simulink model "real_vedio"  (R2021b)
settings: Solver=FixedStepDiscrete  StartTime=0.0  StopTime=100  RelTol=1e-3
PreLoadFcn:
  | n=8; %Number of quantization bits
undefined symbols (not defined in the file): gray, IsPositionTracked, IsSkeletonTracked, JointDepthIndices, JointImageIndices, JointTrackingState, JointWorldCoordinates, none, PositionDepthIndices, PositionImageIndices, PositionWorldCoordinates, Rec, SDTV, SegmentationData, SkeletonTrackingID, videoinput
libraries: commdigbbndpm3 x6, commutil2 x6, dspsigattribs x6, commchan3 x3, visionconversions x2, imaqlib x1
settings Model: Creator=magarini  LastModifiedBy=mluser
settings SolverCC: AlgebraicLoopSolver=TrustRegion
settings DataIOCC: LimitDataPoints=on  SaveFormat=Array  SignalLoggingSaveFormat=ModelDataLogs  ReturnWorkspaceOutputs=off
settings OptimizationCC: BlockReduction=off  ConditionallyExecuteInputs=off  DefaultParameterBehavior=Inlined  ExpressionDepthLimit=2147483647  LifeSpan=inf
settings DebuggingCC: AlgebraicLoopMsg=error  UnderspecifiedInitializationDetection=Classic  MergeDetectMultiDrivingBlocksExec=none  SolverPrmCheckMsg=warning  MultiTaskCondExecSysMsg=warning  MultiTaskRateTransMsg=warning  SingleTaskRateTransMsg=warning  FcnCallInpInsideContextMsg=warning  StateNameClashWarn=warning  SFUnexpectedBacktrackingDiag=warning  SFNoUnconditionalDefaultTransitionDiag=warning  SFExecutionAtInitializationDiag=none  SFMachineParentedDataDiag=warning  ArithmeticOperatorsInVariantConditions=warning
settings HardwareCC: ProdBitPerPointer=32  ProdBitPerSizeT=32  ProdBitPerPtrDiffT=32  ProdLargestAtomicFloat=None  ProdIntDivRoundTo=Undefined  ProdEndianess=Unspecified  ProdWordSize=32  ProdHWDeviceType=ASIC/FPGA->ASIC/FPGA  ProdEqTarget=off
settings ModelReferenceCC: PropagateSignalLabelsOutOfModel=off
settings SFSimCC: SimUseLocalCustomCode=off  SimParseCustomCode=off  CustomCodeUndefinedFunction=UseInterfaceOnly
settings RTWCC: RTWUseLocalCustomCode=off
settings CodeAppCC: StateflowObjectComments=on
settings GRTTargetCC: TargetLangStandard=C89/C90 (ANSI)  CombineOutputUpdateFcns=off  GRTInterface=on
settings ConfigComp: CovMetricSettings=dw  CovSaveCumulativeToWorkspaceVar=on  CovSaveSingleToWorkspaceVar=on  CovExternalEMLEnable=off  CovSFcnEnable=off

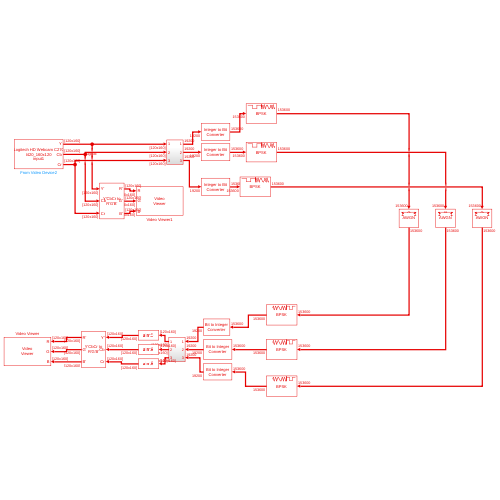
[thumbnail: Simulink's stored preview of the top-level diagram]
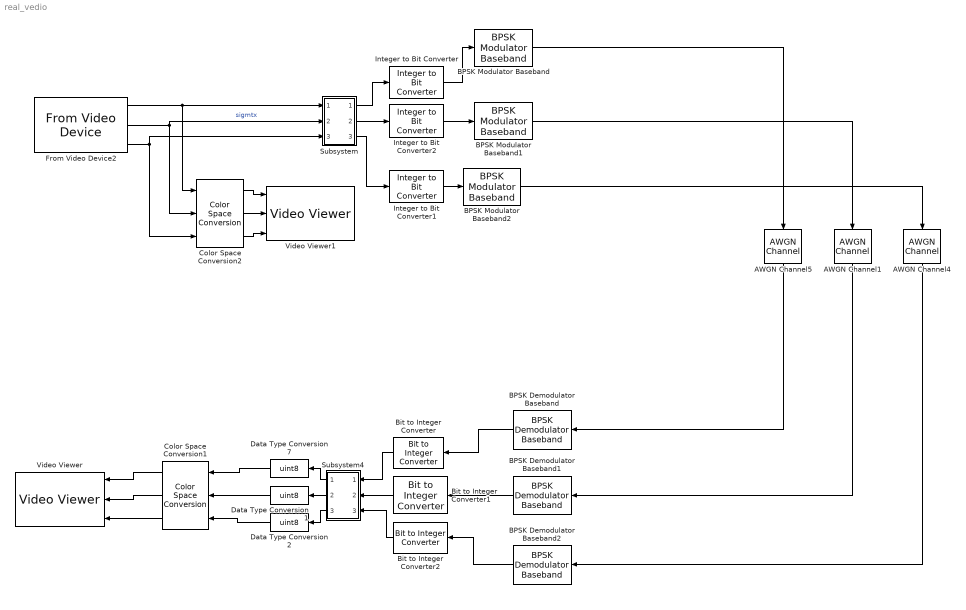
== system real_vedio ==
  AWGN Channel1 : commchan3/AWGN Channel  InputProcessing=Columns as channels (frame based)  seed=67  noiseMode="Signal to noise ratio  (Eb/No)"  EbNodB=10  EsNodB=10  SNRdB=10  bitsPerSym=1  Ps=1  Tsym=1  variance=1
  AWGN Channel4 : commchan3/AWGN Channel  InputProcessing=Columns as channels (frame based)  seed=67  noiseMode="Signal to noise ratio  (Eb/No)"  EbNodB=10  EsNodB=10  SNRdB=10  bitsPerSym=1  Ps=1  Tsym=1  variance=1
  AWGN Channel5 : commchan3/AWGN Channel  InputProcessing=Columns as channels (frame based)  seed=67  noiseMode="Signal to noise ratio  (Eb/No)"  EbNodB=10  EsNodB=10  SNRdB=10  bitsPerSym=1  Ps=1  Tsym=1  variance=1
  BPSK Demodulator Baseband : commdigbbndpm3/BPSK Demodulator Baseband  DecType=Hard decision  VarSource=Dialog  Variance=1  Ph=0  outDtype=Inherit via internal rule  derotateFactorWordLen=16  derotateFactorDataTypeStr=Inherit: Same word length as input  derotateFactorLastDataTypeStr=Inherit: Same word length as input
  BPSK Demodulator Baseband1 : commdigbbndpm3/BPSK Demodulator Baseband  DecType=Hard decision  VarSource=Dialog  Variance=1  Ph=0  outDtype=Inherit via internal rule  derotateFactorWordLen=16  derotateFactorDataTypeStr=Inherit: Same word length as input  derotateFactorLastDataTypeStr=Inherit: Same word length as input
  BPSK Demodulator Baseband2 : commdigbbndpm3/BPSK Demodulator Baseband  DecType=Hard decision  VarSource=Dialog  Variance=1  Ph=0  outDtype=Inherit via internal rule  derotateFactorWordLen=16  derotateFactorDataTypeStr=Inherit: Same word length as input  derotateFactorLastDataTypeStr=Inherit: Same word length as input
  BPSK Modulator Baseband : commdigbbndpm3/BPSK Modulator Baseband  Ph=0  outDtype=double  outWordLen=16  outUDDataType=sfix(16)  outFracLenMode=Best precision  outFracLen=15  outDataTypeStr=double  outLastDataTypeStr=double
  BPSK Modulator Baseband1 : commdigbbndpm3/BPSK Modulator Baseband  Ph=0  outDtype=double  outWordLen=16  outUDDataType=sfix(16)  outFracLenMode=Best precision  outFracLen=15  outDataTypeStr=double  outLastDataTypeStr=double
  BPSK Modulator Baseband2 : commdigbbndpm3/BPSK Modulator Baseband  Ph=0  outDtype=double  outWordLen=16  outUDDataType=sfix(16)  outFracLenMode=Best precision  outFracLen=15  outDataTypeStr=double  outLastDataTypeStr=double
  Bit to Integer Converter : commutil2/Bit to Integer Converter  nbits=8  bitOrder=MSB first  signedOutputValues=Unsigned  outDtype=Inherit via internal rule  outDtypeSigned=Inherit via internal rule
  Bit to Integer Converter1 : commutil2/Bit to Integer Converter  nbits=8  bitOrder=MSB first  signedOutputValues=Unsigned  outDtype=Inherit via internal rule  outDtypeSigned=Inherit via internal rule
  Bit to Integer Converter2 : commutil2/Bit to Integer Converter  nbits=8  bitOrder=MSB first  signedOutputValues=Unsigned  outDtype=Inherit via internal rule  outDtypeSigned=Inherit via internal rule
  Color Space Conversion1 : visionconversions/Color Space  Conversion  conversion=Obsolete  conversionActive=Y'CbCr to R'G'B'  wp_str=D65  rec=Rec. 601 (SDTV)  sys=1125/60/2:1  imagePorts=Separate color signals
  Color Space Conversion2 : visionconversions/Color Space  Conversion  conversion=Obsolete  conversionActive=Y'CbCr to R'G'B'  wp_str=D65  rec=Rec. 601 (SDTV)  sys=1125/60/2:1  imagePorts=Separate color signals
  Data Type Conversion1 : DataTypeConversion  OutDataTypeStr=uint8
  Data Type Conversion2 : DataTypeConversion  OutDataTypeStr=uint8
  Data Type Conversion7 : DataTypeConversion  OutDataTypeStr=uint8
  From Video Device2 : imaqlib/From Video Device  DeviceMenu=INPUTDEVS  Device=winvideo 1 (Logitech HD Webcam C270)  ObjConstructor=videoinput('winvideo', 1)  VideoFormatMenu=INPUTFORMATS  VideoFormat=I420_160x120  VideoSource=input1  ROIPosition=[0 0 120 160]  EnableHWTrigger=off  TriggerConfiguration=none/none  SampleTime=1/25  OutputPortsMode=Separate color signals  DataType=uint8  CanDoHWTrigger=no  ReturnedColorSpace=YCbCr  BlockHandle=5600.0004  ROIWidth=160  ROIHeight=120  ROIColumn=0  ROIRow=0  EngXMLPath=/MATLAB/toolbox/imaq/imaq/private  DevXMLPath=C:\MATLAB\SupportPackages\R2015a\osgenericvideointerface\toolbox\imaq\supportpackages\genericvideo\adaptor\win64  EngLibPath=/MATLAB/toolbox/imaq/imaqblks/imaqmex/glnxa64  ColorSpace=YCbCr  BayerSensorAlignment=grbg  AllMetadata=IsPositionTracked;IsSkeletonTracked;JointDepthIndices;JointImageIndices;JointTrackingState;JointWorldCoordinates;PositionDepthIndices;PositionImageIndices;PositionWorldCoordinates;SegmentationData;SkeletonTrackingID  ImaqMode=off
  Integer to Bit Converter : commutil2/Integer to Bit Converter  nbits=8  signedInputValues=Unsigned  bitOrder=MSB first  outDtype=Inherit via internal rule
  Integer to Bit Converter1 : commutil2/Integer to Bit Converter  nbits=8  signedInputValues=Unsigned  bitOrder=MSB first  outDtype=Inherit via internal rule
  Integer to Bit Converter2 : commutil2/Integer to Bit Converter  nbits=8  signedInputValues=Unsigned  bitOrder=MSB first  outDtype=Inherit via internal rule
  Subsystem : Subsystem
  Subsystem4 : Subsystem
  Video Viewer : VideoViewer  imagePorts=separate color signals  colormapValue=gray(256)  FigPos=[502 1000 410 300]
  Video Viewer1 : VideoViewer  imagePorts=separate color signals  colormapValue=gray(256)  FigPos=[65 1007 410 300]
  wires:
  Color Space Conversion1/1 -> Video Viewer/1
  Color Space Conversion1/2 -> Video Viewer/2
  Color Space Conversion1/3 -> Video Viewer/3
  Color Space Conversion2/1 -> Video Viewer1/1
  Color Space Conversion2/2 -> Video Viewer1/2
  Color Space Conversion2/3 -> Video Viewer1/3
  From Video Device2/2 -> Subsystem/2(In2), Color Space Conversion2/2  "sigmtx"
  From Video Device2/3 -> Subsystem/3(In3), Color Space Conversion2/3
  Subsystem/1(Out1) -> Integer to Bit Converter/1
  Subsystem/2(Out2) -> Integer to Bit Converter2/1
  Subsystem/3(Out3) -> Integer to Bit Converter1/1
  From Video Device2/1 -> Subsystem/1(In1), Color Space Conversion2/1
  Subsystem4/1(Out1) -> Data Type Conversion7/1
  Subsystem4/2(Out2) -> Data Type Conversion1/1
  Subsystem4/3(Out3) -> Data Type Conversion2/1
  BPSK Demodulator Baseband/1 -> Bit to Integer Converter/1
  BPSK Demodulator Baseband1/1 -> Bit to Integer Converter1/1
  BPSK Demodulator Baseband2/1 -> Bit to Integer Converter2/1
  Integer to Bit Converter/1 -> BPSK Modulator Baseband/1
  Integer to Bit Converter1/1 -> BPSK Modulator Baseband2/1
  Integer to Bit Converter2/1 -> BPSK Modulator Baseband1/1
  Bit to Integer Converter/1 -> Subsystem4/1(In1)
  Bit to Integer Converter1/1 -> Subsystem4/2(In2)
  Bit to Integer Converter2/1 -> Subsystem4/3(In3)
  Data Type Conversion7/1 -> Color Space Conversion1/1
  Data Type Conversion1/1 -> Color Space Conversion1/2
  Data Type Conversion2/1 -> Color Space Conversion1/3
  BPSK Modulator Baseband/1 -> AWGN Channel5/1
  BPSK Modulator Baseband1/1 -> AWGN Channel1/1
  BPSK Modulator Baseband2/1 -> AWGN Channel4/1
  AWGN Channel5/1 -> BPSK Demodulator Baseband/1
  AWGN Channel1/1 -> BPSK Demodulator Baseband1/1
  AWGN Channel4/1 -> BPSK Demodulator Baseband2/1

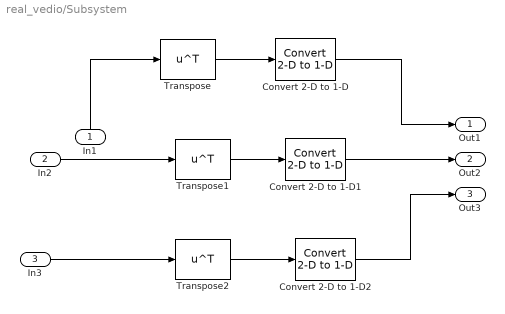
== system real_vedio/Subsystem ==
  In1 : Inport
  In2 : Inport  Port=2
  In3 : Inport  Port=3
  Convert 2-D to 1-D : dspsigattribs/Convert 2-D to 1-D
      settings: SourceProductBaseCode=DS
  Convert 2-D to 1-D1 : dspsigattribs/Convert 2-D to 1-D
      settings: SourceProductBaseCode=DS
  Convert 2-D to 1-D2 : dspsigattribs/Convert 2-D to 1-D
      settings: SourceProductBaseCode=DS
  Transpose : Math  Operator=transpose  SignedPower=on  SaturateOnIntegerOverflow=on
  Transpose1 : Math  Operator=transpose  SignedPower=on  SaturateOnIntegerOverflow=on
  Transpose2 : Math  Operator=transpose  SignedPower=on  SaturateOnIntegerOverflow=on
  Out1 : Outport
  Out2 : Outport  Port=2
  Out3 : Outport  Port=3
  wires:
  In3/1 -> Transpose2/1
  In2/1 -> Transpose1/1
  In1/1 -> Transpose/1
  Transpose2/1 -> Convert 2-D to 1-D2/1
  Transpose1/1 -> Convert 2-D to 1-D1/1
  Transpose/1 -> Convert 2-D to 1-D/1
  Convert 2-D to 1-D2/1 -> Out3/1
  Convert 2-D to 1-D1/1 -> Out2/1
  Convert 2-D to 1-D/1 -> Out1/1

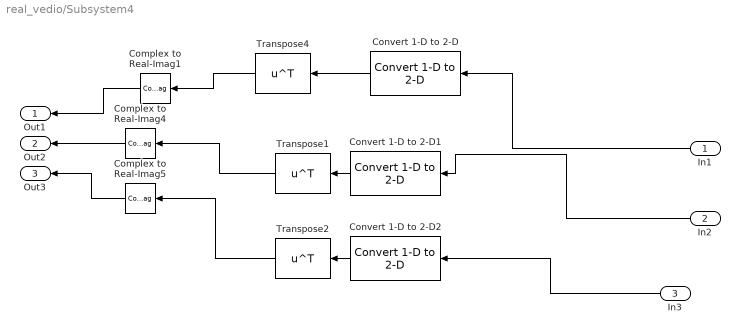
== system real_vedio/Subsystem4 ==
  In1 : Inport
  In2 : Inport  Port=2
  In3 : Inport  Port=3
  Complex to Real-Imag1 : ComplexToRealImag  Output=Real
  Complex to Real-Imag4 : ComplexToRealImag  Output=Real
  Complex to Real-Imag5 : ComplexToRealImag  Output=Real
  Convert 1-D to 2-D : dspsigattribs/Convert 1-D to 2-D  M=160  N=120  frameBasedOut=off
      settings: SourceProductBaseCode=DS
  Convert 1-D to 2-D1 : dspsigattribs/Convert 1-D to 2-D  M=160  N=120  frameBasedOut=off
      settings: SourceProductBaseCode=DS
  Convert 1-D to 2-D2 : dspsigattribs/Convert 1-D to 2-D  M=160  N=120  frameBasedOut=off
      settings: SourceProductBaseCode=DS
  Transpose1 : Math  Operator=transpose  SignedPower=on  OutputSignalType=complex  SaturateOnIntegerOverflow=on
  Transpose2 : Math  Operator=transpose  SignedPower=on  OutputSignalType=complex  SaturateOnIntegerOverflow=on
  Transpose4 : Math  Operator=transpose  SignedPower=on  OutputSignalType=complex  SaturateOnIntegerOverflow=on
  Out1 : Outport
  Out2 : Outport  Port=2
  Out3 : Outport  Port=3
  wires:
  Transpose2/1 -> Complex to Real-Imag5/1
  Transpose4/1 -> Complex to Real-Imag1/1
  In1/1 -> Convert 1-D to 2-D/1
  In2/1 -> Convert 1-D to 2-D1/1
  In3/1 -> Convert 1-D to 2-D2/1
  Convert 1-D to 2-D/1 -> Transpose4/1
  Transpose1/1 -> Complex to Real-Imag4/1
  Convert 1-D to 2-D1/1 -> Transpose1/1
  Convert 1-D to 2-D2/1 -> Transpose2/1
  Complex to Real-Imag4/1 -> Out2/1
  Complex to Real-Imag5/1 -> Out3/1
  Complex to Real-Imag1/1 -> Out1/1
